simulink model "spcomm2"  (R2014a)
settings: Solver=ode45  StartTime=0.0  StopTime=0.05  RelTol=1e-3
values from neighbouring files (symbols this model uses):
  ch_delay = 12.4    [spcomm_ini.m]
  deltaT_per_sample = bit_clk_err_ratio    (= 0.0001)    [spcomm_ini.m]
  f_err = 100    [spcomm_ini.m]
  rolloff = 0.25    [spcomm_ini.m]
  rrc_multiply_rate = 4    [spcomm_ini.m]
  rrc_span_symbol = 16    [spcomm_ini.m]
  sp_factor = 256    [spcomm_ini.m]
  tao1 = Kvco/(wn^2)    (= 122.230996295)    [spcomm_ini.m]
  tao2 = Ksai*2/wn    (= 0.00318309886184)    [spcomm_ini.m]
  Tb = 1/bit_rate    (= 0.000133333333333)    [spcomm_ini.m]
  Ts = 1/bit_rate/sp_factor/rrc_multiply_rate    (= 1.30208333333e-07)    [spcomm_ini.m]
  Tspb = 1/bit_rate/sp_factor    (= 5.20833333333e-07)    [spcomm_ini.m]
undefined symbols (not defined in the file or in its folder): dfilt, DiscIntNeverNeededParam, magnitude
libraries: dspsigops x3, commfilt2 x3, dsparch4 x2, commnoisgen2 x1, simulink x1
settings Model: Creator=dell  LastModifiedBy=chenpeng

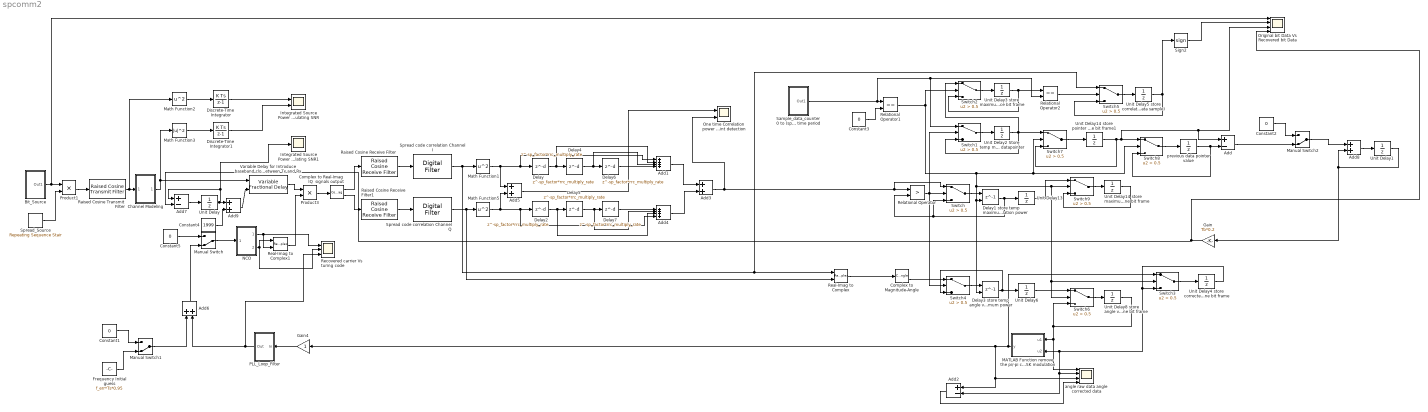
== system spcomm2 ==
  Add : Sum  Inputs=+-
  Add1 : Sum  Inputs=++++
  Add2 : Sum  Inputs=+-
  Add{3,5..6,8..9} (5 alike) : Sum
  Add4 : Sum  Inputs=++++
  Add7 : Sum  Inputs=+-
  Bit_Source : Subsystem
  Channel Modeling : Subsystem
  Complex to Magnitude-Angle : ComplexToMagnitudeAngle
  Complex to Real-Imag IQ  signals output : ComplexToRealImag
  Constant{1..3,5} (4 alike) : Constant  Value=0
  Constant4 : Constant  Value=1999
  Delay{,2,4..7} (6 alike) : Delay  DelayLength=sp_factor*rrc_multiply_rate
  Delay1 store temp maximum correlation power : Delay  DelayLength=1  ExternalReset=Rising  InputProcessing=Columns as channels (frame based)
      settings: InputPortMap=u0,r5
  Delay3 store temp angle value at temp maximum power : Delay  DelayLength=1  ExternalReset=Rising  InputProcessing=Columns as channels (frame based)
      settings: InputPortMap=u0,r5
  Discrete-Time Integrator : DiscreteIntegrator  SampleTime=-1  ICPrevOutput=DiscIntNeverNeededParam  ICPrevScaledInput=DiscIntNeverNeededParam
  Discrete-Time Integrator1 : DiscreteIntegrator  SampleTime=-1  ICPrevOutput=DiscIntNeverNeededParam  ICPrevScaledInput=DiscIntNeverNeededParam
  Frequency Initial guess : Constant  Value=f_err*Ts*0.95
  Gain : Gain  Gain=Tb*0.2
  Gain4 : Gain  SampleTime=Tb
  Integrated Source Power and Noise Power for Calculating SNR : Scope  NumInputPorts=2
      settings: YMin=0~0  YMax=0.00475~5.25  SaveName=ScopeData2
  Integrated Source Power and Noise Power for Calculating SNR1 : Scope
      settings: YMin=-13  YMax=0  SaveName=ScopeData6
  MATLAB Function remove the pi/-pi caused by BPSK modulation : MATLAB Function  TreatAsAtomicUnit=on
  Manual Switch : ManualSwitch  CurrentSetting=0
  Manual Switch1 : ManualSwitch  CurrentSetting=0
  Manual Switch2 : ManualSwitch  CurrentSetting=0
  Math Function1 : Math  Operator=square  SaturateOnIntegerOverflow=on
  Math Function2 : Math  Operator=square  SaturateOnIntegerOverflow=on
  Math Function3 : Math  Operator=magnitude^2  SaturateOnIntegerOverflow=on
  Math Function5 : Math  Operator=square  SaturateOnIntegerOverflow=on
  NCO : Subsystem
  One time Correlation power Vs four time Correlation power for improve data start point detection : Scope  NumInputPorts=2
      settings: YMin=0~0  YMax=85000~300000  SaveName=ScopeData4
  Original bit Data Vs Recovered bit Data : Scope  NumInputPorts=4
      settings: YMin=-1~0~0~0  YMax=1~5.25~1100~0.00011  SaveName=ScopeData3
  PLL_Loop_Filter : Subsystem
  Product1 : Product  SampleTime=Tspb
  Product3 : Product
  Raised Cosine Receive Filter : commfilt2/Raised Cosine Receive Filter  filtType=Square root  N=rrc_multiply_rate  filtSpan=rrc_span_symbol  currentFiltSpan=rrc_span_symbol  D=(rrc_span_symbol)/2  R=rolloff  sampMode=Mute  saveAsFlag=0  rateMode=Downsampling  downFactor=1  downOffset=0  framing=Enforce single-rate processing  InputProcessing=Columns as channels (frame based)  checkGain=Normalized  filterGain=1  checkCoeff=off  variableName=rcRxFilt  launchFVT=on  roundingMode=Floor  overflowMode=off
  Raised Cosine Receive Filter1 : commfilt2/Raised Cosine Receive Filter  filtType=Square root  N=rrc_multiply_rate  filtSpan=rrc_span_symbol  currentFiltSpan=rrc_span_symbol  D=(rrc_span_symbol)/2  R=rolloff  sampMode=Mute  saveAsFlag=0  rateMode=Downsampling  downFactor=1  downOffset=0  framing=Enforce single-rate processing  InputProcessing=Columns as channels (frame based)  checkGain=Normalized  filterGain=1  checkCoeff=off  variableName=rcRxFilt1  launchFVT=on  roundingMode=Floor  overflowMode=off
  Raised Cosine Transmit Filter : commfilt2/Raised Cosine Transmit Filter  filtType=Square root  filtSpan=rrc_span_symbol  currentFiltSpan=16  D=(16)/2  R=rolloff  sampMode=Mute  saveAsFlag=0  N=rrc_multiply_rate  framing=Allow multirate processing  checkGain=Normalized  filterGain=1  checkCoeff=off  variableName=rcTxFilt1  launchFVT=on  roundingMode=Floor  overflowMode=off
  Real-Imag to Complex : RealImagToComplex
  Real-Imag to Complex1 : RealImagToComplex
  Recovered carrier Vs turing code : Scope  NumInputPorts=3
      settings: TimeRange=0.01  YMin=-1~-1~6.51e-07  YMax=-0.05~0.7~6.545e-07  MaxDataPoints=200000
  Relational Operator : RelationalOperator  Operator=>  OutDataTypeStr=boolean
  Relational Operator1 : RelationalOperator  Operator===  OutDataTypeStr=boolean
  Relational Operator2 : RelationalOperator  Operator===  OutDataTypeStr=boolean
  Sample_data_counter 0 to (sp_factor*upconversion_rate-1) count every Ts time period : Subsystem
  Sign2 : Signum
  Spread code correlation Channel I : dsparch4/Digital Filter  TypePopup=FIR (all zeros)  IIRFiltStruct=Direct form II transposed  AllPoleFiltStruct=Direct form  FIRFiltStruct=Direct form  CoeffSource=Specify via dialog  NumCoeffs=spread_code_up  DenCoeffs=[1 0.1]  BiQuadCoeffs=[1 0.3 0.4 1 0.1 0.2]  LatticeCoeffs=[0.2 0.4]  denIgnore=on  FiltPerSampPopup=One filter per frame  IC=0  ICnum=0  ICden=0  roundingMode=Floor  overflowMode=off  ScaleValues=1  scaleValueFracLength=14  stageInFracLength=15  stageOutFracLength=15  FilterSource=Specify via dialog  dfiltObjectName=dfilt.dffir([1 2 1])  InputProcessing=Columns as channels (frame based)
  Spread code correlation Channel Q : dsparch4/Digital Filter  TypePopup=FIR (all zeros)  IIRFiltStruct=Direct form II transposed  AllPoleFiltStruct=Direct form  FIRFiltStruct=Direct form  CoeffSource=Specify via dialog  NumCoeffs=spread_code_up  DenCoeffs=[1 0.1]  BiQuadCoeffs=[1 0.3 0.4 1 0.1 0.2]  LatticeCoeffs=[0.2 0.4]  denIgnore=on  FiltPerSampPopup=One filter per frame  IC=0  ICnum=0  ICden=0  roundingMode=Floor  overflowMode=off  ScaleValues=1  scaleValueFracLength=14  stageInFracLength=15  stageOutFracLength=15  FilterSource=Specify via dialog  dfiltObjectName=dfilt.dffir([1 2 1])  InputProcessing=Columns as channels (frame based)
  Spread_Source : simulink/Sources/Repeating Sequence Stair  OutValues=spread_code'  tsamp=Tspb  OutMin=[]  OutMax=[]  OutDataTypeStr=double  OutputDataTypeScalingMode=double  OutDataType=fixdt(0,8)  ConRadixGroup=Best Precision: Vector-wise  OutScaling=2^-12
  Switch{,1..9} (10 alike) : Switch  Criteria=u2 > Threshold  Threshold=0.5
  Unit Delay : UnitDelay  SampleTime=Ts
  Unit Delay1 : UnitDelay  SampleTime=Tb
  Unit Delay13 : UnitDelay  SampleTime=-1
  Unit Delay14 store maximum correlation power at one bit frame : UnitDelay  SampleTime=-1
  Unit Delay14 store pointer at one bit frame1 : UnitDelay  SampleTime=-1
  Unit Delay2 Store temp maximum datapointer : UnitDelay  SampleTime=-1
  Unit Delay3 store maximum datapointer for one source bit frame : UnitDelay  SampleTime=-1
  Unit Delay4 store corrected angle value at maximum power for one bit frame : UnitDelay  SampleTime=-1
  Unit Delay5 store correlate data sample at datapointer time (recovered data sample) : UnitDelay  SampleTime=-1
  Unit Delay6 : UnitDelay  SampleTime=-1
  Unit Delay8 store angle value at maximum power for one bit frame : UnitDelay  SampleTime=-1
  "Variable Delay for Introduce baseband clock error between Tx and Rx " : dspsigops/Variable Fractional Delay  mode=OBSOLETE  modeActive=Linear  dmax=2000  InputProcessing=Columns as channels (frame based)  L=4  FarrowL=4  R=10  alpha=1  ic=0  fallbackFIR=Clip to the minimum value necessary for centered kernel  fallbackFarrow=Clip to the minimum value necessary for centered kernel  noDFT=off  roundingMode=Zero  overflowMode=off
  angle raw data angle corrected data : Scope  NumInputPorts=4
      settings: YMin=-3.5~-3.5~-3.5~-5.5  YMax=3.5~6~6~3
  previous data pointer value : UnitDelay  SampleTime=-1
  wires:
  Product1/1 -> Raised Cosine Transmit Filter/1
  Spread_Source/1 -> Product1/2
  Relational Operator/1 -> Switch/2, Switch1/2, Switch4/2
  Switch/1 -> Delay1 store temp maximum correlation power/1
  Switch1/1 -> Unit Delay2 Store temp maximum datapointer/1
  Constant3/1 -> Relational Operator1/2
  Relational Operator1/1 -> Switch2/2, Switch8/2, Switch7/2, Switch3/2, Switch6/2, Switch9/2, Delay3 store temp angle value at temp maximum power/2, Delay1 store temp maximum correlation power/2
  Delay1 store temp maximum correlation power/1 -> Unit Delay13/1, Relational Operator/2, Switch/3
  Switch2/1 -> Unit Delay3 store maximum datapointer for one source bit frame/1
  Unit Delay2 Store temp maximum datapointer/1 -> Switch7/1, Switch1/3, Switch2/1
  Unit Delay3 store maximum datapointer for one source bit frame/1 -> Relational Operator2/1, Switch2/3
  Switch9/1 -> Unit Delay14 store maximum correlation power at one bit frame/1
  Unit Delay14 store maximum correlation power at one bit frame/1 -> Switch9/3
  Unit Delay13/1 -> Switch9/1
  Add3/1 -> One time Correlation power Vs four time Correlation power for improve data start point detection/2, Relational Operator/1, Switch/1
  Real-Imag to Complex/1 -> Complex to Magnitude-Angle/1
  Delay3 store temp angle value at temp maximum power/1 -> Unit Delay6/1, Switch4/3
  Switch4/1 -> Delay3 store temp angle value at temp maximum power/1
  Complex to Magnitude-Angle/2 -> Switch4/1
  Unit Delay8 store angle value at maximum power for one bit frame/1 -> Switch6/3, angle raw data angle corrected data/1, MATLAB Function remove the pi/-pi caused by BPSK modulation/1(u1)
  Unit Delay6/1 -> Switch6/1
  Switch6/1 -> Unit Delay8 store angle value at maximum power for one bit frame/1
  Spread code correlation Channel I/1 -> Real-Imag to Complex/1, Switch5/1, Math Function1/1
  Spread code correlation Channel Q/1 -> Real-Imag to Complex/2, Math Function5/1
  Bit_Source/1(Out1) -> Original bit Data Vs Recovered bit Data/1, Product1/1
  Raised Cosine Transmit Filter/1 -> Math Function2/1, Channel Modeling/1(In1)
  Raised Cosine Receive Filter/1 -> Spread code correlation Channel I/1
  Raised Cosine Receive Filter1/1 -> Spread code correlation Channel Q/1
  NCO/1(Sin) -> Recovered carrier Vs turing code/1, Real-Imag to Complex1/2
  NCO/2(Cos) -> Recovered carrier Vs turing code/2, Real-Imag to Complex1/1
  Channel Modeling/1(Out1) -> "Variable Delay for Introduce baseband clock error between Tx and Rx "/1, Math Function3/1
  Real-Imag to Complex1/1 -> Product3/2
  Product3/1 -> Complex to Real-Imag IQ  signals output/1
  Complex to Real-Imag IQ  signals output/1 -> Raised Cosine Receive Filter/1
  Complex to Real-Imag IQ  signals output/2 -> Raised Cosine Receive Filter1/1
  Manual Switch/1 -> NCO/1(Freq)
  Gain4/1 -> PLL_Loop_Filter/1(In)
  PLL_Loop_Filter/1(Out) -> Add6/2, Recovered carrier Vs turing code/3
  Math Function1/1 -> Add1/1, Delay/1, Add5/1
  Math Function5/1 -> Add4/4, Delay2/1, Add5/2
  Delay/1 -> Add1/2, Delay4/1
  Delay4/1 -> Add1/3, Delay6/1
  Delay2/1 -> Add4/3, Delay5/1
  Delay5/1 -> Add4/2, Delay7/1
  Math Function2/1 -> Discrete-Time Integrator/1
  Math Function3/1 -> Discrete-Time Integrator1/1
  Discrete-Time Integrator1/1 -> Integrated Source Power and Noise Power for Calculating SNR/2
  Discrete-Time Integrator/1 -> Integrated Source Power and Noise Power for Calculating SNR/1
  Delay6/1 -> Add1/4
  Delay7/1 -> Add4/1
  Add1/1 -> Add3/1
  Add4/1 -> Add3/2
  Switch3/1 -> Unit Delay4 store corrected angle value at maximum power for one bit frame/1
  Unit Delay4 store corrected angle value at maximum power for one bit frame/1 -> Add2/2, angle raw data angle corrected data/2, MATLAB Function remove the pi/-pi caused by BPSK modulation/2(u2), Switch3/3
  MATLAB Function remove the pi/-pi caused by BPSK modulation/1(y) -> Switch3/1, Add2/1, angle raw data angle corrected data/3, Gain4/1
  Relational Operator2/1 -> Switch5/2
  Switch5/1 -> Unit Delay5 store correlate data sample at datapointer time (recovered data sample)/1
  Unit Delay5 store correlate data sample at datapointer time (recovered data sample)/1 -> Switch5/3, Sign2/1
  Sign2/1 -> Original bit Data Vs Recovered bit Data/2
  Sample_data_counter 0 to (sp_factor*upconversion_rate-1) count every Ts time period/1(Out1) -> Relational Operator2/2, Switch1/1, Relational Operator1/1
  Add5/1 -> One time Correlation power Vs four time Correlation power for improve data start point detection/1
  Constant5/1 -> Manual Switch/1
  Add6/1 -> Manual Switch/2
  Add2/1 -> angle raw data angle corrected data/4
  Constant1/1 -> Manual Switch1/1
  Frequency Initial guess/1 -> Manual Switch1/2
  Manual Switch1/1 -> Add6/1
  Switch7/1 -> Unit Delay14 store pointer at one bit frame1/1
  Unit Delay14 store pointer at one bit frame1/1 -> Original bit Data Vs Recovered bit Data/3, Add/1, Switch8/1, Switch7/3
  Switch8/1 -> previous data pointer value/1
  previous data pointer value/1 -> Add/2, Switch8/3
  Add7/1 -> Unit Delay/1
  Unit Delay/1 -> Integrated Source Power and Noise Power for Calculating SNR1/1, Add7/1, Add9/1
  "Variable Delay for Introduce baseband clock error between Tx and Rx "/1 -> Product3/1
  Add8/1 -> Unit Delay1/1
  Unit Delay1/1 -> Gain/1, Add8/2
  Gain/1 -> Add7/2, Original bit Data Vs Recovered bit Data/4
  Constant2/1 -> Manual Switch2/1
  Add9/1 -> "Variable Delay for Introduce baseband clock error between Tx and Rx "/2
  Constant4/1 -> Add9/2
  Add/1 -> Manual Switch2/2
  Manual Switch2/1 -> Add8/1

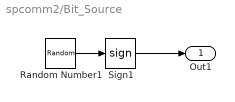
== system spcomm2/Bit_Source ==
  Random Number1 : RandomNumber  Seed=157  SampleTime=Tb
  Sign1 : Signum
  Out1 : Outport
  wires:
  Sign1/1 -> Out1/1
  Random Number1/1 -> Sign1/1

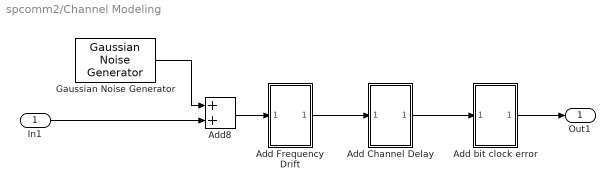
== system spcomm2/Channel Modeling ==
  In1 : Inport
  Add Channel Delay : Subsystem
  Add Frequency Drift : Subsystem
  Add bit clock error : Subsystem
  Add8 : Sum
  Gaussian Noise Generator : commnoisgen2/Gaussian Noise Generator  m=0  d=1  s=41  Ts=Ts  frameBased=off  sampPerFrame=1  orient=off  outDataType=double
  Out1 : Outport
  wires:
  In1/1 -> Add8/2
  Gaussian Noise Generator/1 -> Add8/1
  Add Channel Delay/1(Out1) -> Add bit clock error/1(In1)
  Add bit clock error/1(Out1) -> Out1/1
  Add8/1 -> Add Frequency Drift/1(In1)
  Add Frequency Drift/1(Out1) -> Add Channel Delay/1(In1)

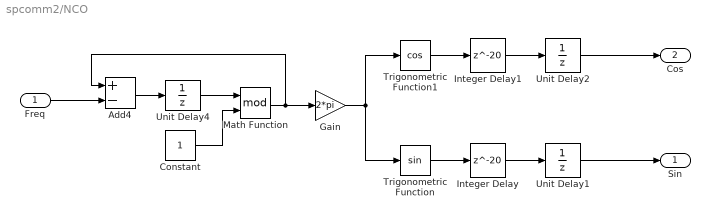
== system spcomm2/NCO ==
  Freq : Inport
  Add4 : Sum  Inputs=+-
  Constant : Constant
  Gain : Gain  Gain=2*pi
  Integer Delay : Delay  DelayLength=20  InputProcessing=Inherited
  Integer Delay1 : Delay  DelayLength=20  InputProcessing=Inherited
  Math Function : Math  Operator=mod  SaturateOnIntegerOverflow=on
  Trigonometric Function : Trigonometry
  Trigonometric Function1 : Trigonometry  Operator=cos
  Unit Delay1 : UnitDelay  SampleTime=-1
  Unit Delay2 : UnitDelay  SampleTime=-1
  Unit Delay4 : UnitDelay  SampleTime=Ts
  Sin : Outport
  Cos : Outport  Port=2
  wires:
  Gain/1 -> Trigonometric Function/1, Trigonometric Function1/1
  Trigonometric Function/1 -> Integer Delay/1
  Trigonometric Function1/1 -> Integer Delay1/1
  Unit Delay1/1 -> Sin/1
  Unit Delay2/1 -> Cos/1
  Integer Delay/1 -> Unit Delay1/1
  Integer Delay1/1 -> Unit Delay2/1
  Add4/1 -> Unit Delay4/1
  Unit Delay4/1 -> Math Function/1
  Math Function/1 -> Gain/1, Add4/1
  Constant/1 -> Math Function/2
  Freq/1 -> Add4/2

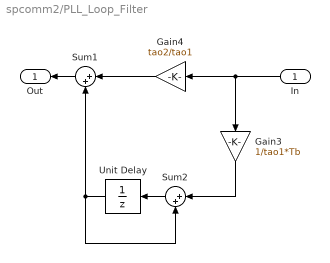
== system spcomm2/PLL_Loop_Filter ==
  In : Inport
  Gain3 : Gain  Gain=1/tao1*Tb  SampleTime=Tb
  Gain4 : Gain  Gain=tao2/tao1  SampleTime=Tb
  Sum1 : Sum  Inputs=|++
  Sum2 : Sum  Inputs=|++
  Unit Delay : UnitDelay  SampleTime=Tb
  Out : Outport
  wires:
  In/1 -> Gain4/1, Gain3/1
  Sum1/1 -> Out/1
  Sum2/1 -> Unit Delay/1
  Unit Delay/1 -> Sum1/2, Sum2/2
  Gain3/1 -> Sum2/1
  Gain4/1 -> Sum1/1

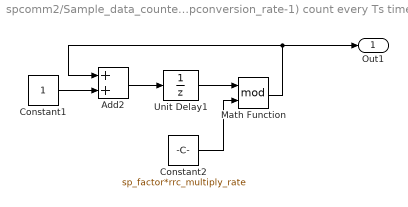
== system spcomm2/Sample_data_counter 0 to (sp_factor*upconversion_rate-1) count every Ts time period ==
  Add2 : Sum  SampleTime=1/bit_rate/sp_factor/rrc_multiply_rate
  Constant1 : Constant
  Constant2 : Constant  Value=sp_factor*rrc_multiply_rate
  Math Function : Math  Operator=mod  SaturateOnIntegerOverflow=on
  Unit Delay1 : UnitDelay  SampleTime=-1
  Out1 : Outport
  wires:
  Constant1/1 -> Add2/2
  Math Function/1 -> Out1/1, Add2/1
  Constant2/1 -> Math Function/2
  Add2/1 -> Unit Delay1/1
  Unit Delay1/1 -> Math Function/1

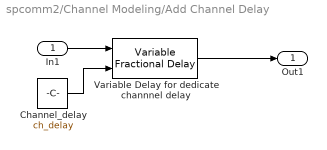
== system spcomm2/Channel Modeling/Add Channel Delay ==
  In1 : Inport
  Channel_delay : Constant  Value=ch_delay
  Variable Delay for dedicate channnel delay : dspsigops/Variable Fractional Delay  mode=OBSOLETE  modeActive=Farrow  dmax=100  InputProcessing=Columns as channels (frame based)  L=4  FarrowL=4  R=10  alpha=1  ic=0  fallbackFIR=Clip to the minimum value necessary for centered kernel  fallbackFarrow=Clip to the minimum value necessary for centered kernel  noDFT=off  roundingMode=Zero  overflowMode=off
  Out1 : Outport
  wires:
  Channel_delay/1 -> Variable Delay for dedicate channnel delay/2
  In1/1 -> Variable Delay for dedicate channnel delay/1
  Variable Delay for dedicate channnel delay/1 -> Out1/1

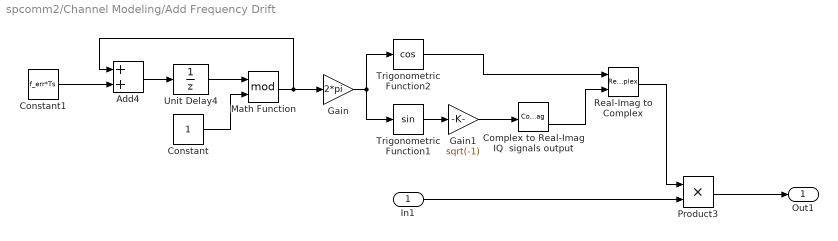
== system spcomm2/Channel Modeling/Add Frequency Drift ==
  In1 : Inport
  Add4 : Sum
  Complex to Real-Imag IQ  signals output : ComplexToRealImag
  Constant : Constant
  Constant1 : Constant  Value=f_err*Ts
  Gain : Gain  Gain=2*pi
  Gain1 : Gain  Gain=sqrt(-1)
  Math Function : Math  Operator=mod  SaturateOnIntegerOverflow=on
  Product3 : Product
  Real-Imag to Complex : RealImagToComplex
  Trigonometric Function1 : Trigonometry
  Trigonometric Function2 : Trigonometry  Operator=cos
  Unit Delay4 : UnitDelay  SampleTime=Ts
  Out1 : Outport
  wires:
  In1/1 -> Product3/2
  Add4/1 -> Unit Delay4/1
  Product3/1 -> Out1/1
  Unit Delay4/1 -> Math Function/1
  Math Function/1 -> Gain/1, Add4/1
  Constant/1 -> Math Function/2
  Constant1/1 -> Add4/2
  Gain/1 -> Trigonometric Function1/1, Trigonometric Function2/1
  Trigonometric Function1/1 -> Gain1/1
  Trigonometric Function2/1 -> Real-Imag to Complex/1
  Real-Imag to Complex/1 -> Product3/1
  Gain1/1 -> Complex to Real-Imag IQ  signals output/1
  Complex to Real-Imag IQ  signals output/2 -> Real-Imag to Complex/2

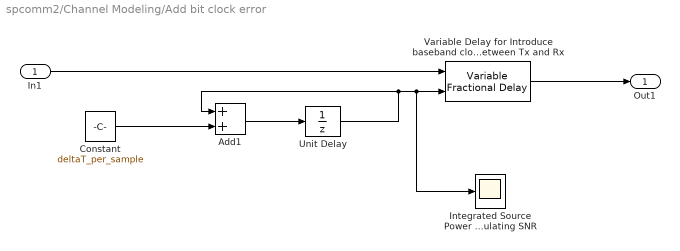
== system spcomm2/Channel Modeling/Add bit clock error ==
  In1 : Inport
  Add1 : Sum
  Constant : Constant  Value=deltaT_per_sample
  Integrated Source Power and Noise Power for Calculating SNR : Scope
      settings: YMin=0  YMax=15  SaveName=ScopeData5
  Unit Delay : UnitDelay  SampleTime=Ts
  "Variable Delay for Introduce baseband clock error between Tx and Rx " : dspsigops/Variable Fractional Delay  mode=OBSOLETE  modeActive=Linear  dmax=2000  InputProcessing=Columns as channels (frame based)  L=4  FarrowL=4  R=10  alpha=1  ic=0  fallbackFIR=Clip to the minimum value necessary for centered kernel  fallbackFarrow=Clip to the minimum value necessary for centered kernel  noDFT=off  roundingMode=Zero  overflowMode=off
  Out1 : Outport
  wires:
  "Variable Delay for Introduce baseband clock error between Tx and Rx "/1 -> Out1/1
  Add1/1 -> Unit Delay/1
  In1/1 -> "Variable Delay for Introduce baseband clock error between Tx and Rx "/1
  Constant/1 -> Add1/2
  Unit Delay/1 -> Integrated Source Power and Noise Power for Calculating SNR/1, "Variable Delay for Introduce baseband clock error between Tx and Rx "/2, Add1/1

== matlab function spcomm2/MATLAB Function remove the pi//-pi caused by BPSK modulation ==
  data: u1 input; y output; u2 input
function y = fcn(u1,u2)
%#codegen
if (u1-u2) > pi/2
    y = u1-pi;
else
    if (u1-u2)<-pi/2
        y = u1+pi;
    else
        y = u1;
    end;
end;
